simulink model "test"  (R2022b)
settings: Solver=VariableStepAuto  StartTime=0.0  StopTime=20  RelTol=1e-3
values from neighbouring files (symbols this model uses):
  N = 3    [kuka_IMPC_PriController_simulink_initial.m]
undefined symbols (not defined in the file or in its folder): DiscIntNeverNeededParam, exJoint, t_max
libraries: simulink x1, cstblocks x1, cjt_library_models x1
settings Model: Creator=zheng  LastModifiedBy=zheng
settings ModelReferenceCC: EnableRefExpFcnMdlSchedulingChecks=on

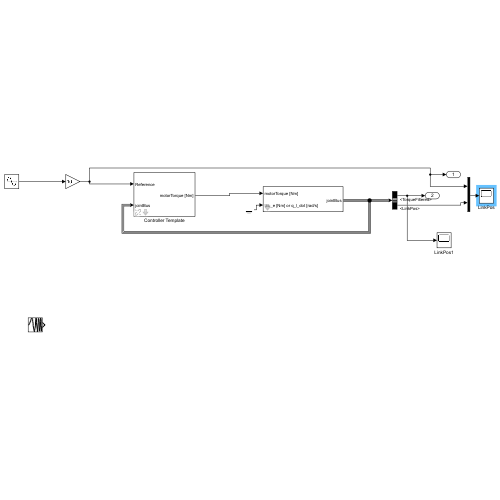
[thumbnail: Simulink's stored preview of the top-level diagram]
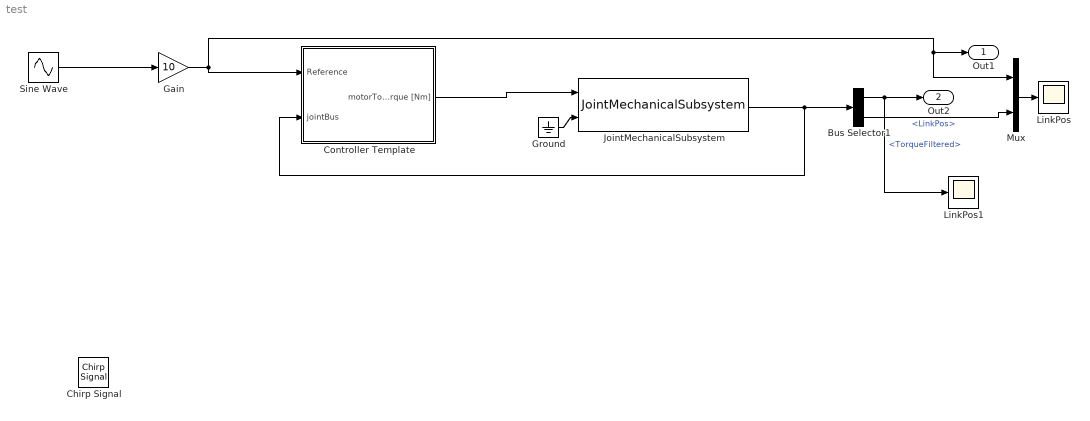
== system test ==
  Bus Selector1 : BusSelector  OutputSignals=TorqueFiltered,LinkPos
  Chirp Signal : simulink/Sources/Chirp Signal  f1=f_min  T=t_max  f2=f_max
  Controller Template : Subsystem  AncestorBlock=cjt_library_controllers/Controllers/Controller Template  mask(CJT Controller Template){jointObj=exJoint}
      mask prompts: jointObj "Joint Object"
      mask help:
      | This is a template block. If you have a controller that you wish to contribute to this library, this block here  represents your interface.
      |
      | Here are the steps to contribute your controller using this template:
      |
      | 1. Copy this block into your development. Disable and break its link to this library. You now have a copy of the interface in your model that is disconnected from the library.
      |
      | 2. Implement your controller within this block. The controller should use no hardcoded values. Wherever you can, access the properties of a CJT joint object. The joint object should be passed to the block through the mask as first parameter (e.g. jointObj).
      |
      | 3. Complete the block mask, so the user can specify all block properties programatically or manually through the mask.
      |
      | 4. Make an example:
      | a) Clean your development model up and convert it into a minimum example that demonstrates the use of your block.
      | b) Create an m-script that configures the required joint object and simulation parameters, runs the model.and displays some results. See existing examples and copy their format.
      | c) Write the documentation of your block.
      |
      | 5. Write a unit test. Look into the unit test directory and open the unit test file for this library. Add a test for your block. A good point to start is your example. Make the test pass.
      |
      | 6. Submit your contribution!
      |
      | Thanks a lot!
      |
      | 7.
      mask init:
      | % Do all the controller related computations here.
      | % Compute gains etc.
      | 
      | % E.g. get linear dynamics matrices first...
      | [A, B, C, I, D, K] = jointObj.getDynamicsMatrices();
      | 
      | % YOUR CODE HERE
      settings: LibrarySourceBlock=cjt_library_controllers/Controllers/Controller Template
      mask Help:
      | This is a template block. If you have a controller that you wish to contribute to this library, this block here  represents your interface.
      | 
      | Here are the steps to contribute your controller using this template:
      | 
      | 1. Copy this block into your development. Disable and break its link to this library. You now have a copy of the interface in your model that is disconnected from the library.
      | 
      | 2. Implement your controller within this block. The controller should use no hardcoded values. Wherever you can, access the properties of a CJT joint object. The joint object should be passed to the block through the mask as first parameter (e.g. jointObj).
      | 
      | 3. Complete the block mask, so the user can specify all block properties programatically or manually through the mask.
      | 
      | 4. Make an example:
      | a) Clean your development model up and convert it into a minimum example that demonstrates the use of your block.
      | b) Create an m-script that configures the required joint object and simulation parameters, runs the model.and displays some results. See existing examples and copy their format.
      | c) Write the documentation of your block.
      | 
      | 5. Write a unit test. Look into the unit test directory and open the unit test file for this library. Add a test for your block. A good point to start is your example. Make the test pass.
      | 
      | 6. Submit your contribution!
      | 
      | Thanks a lot!
  Gain : Gain  Gain=10
  Ground : Ground
  JointMechanicalSubsystem : cjt_library_models/Joint models/JointMechanicalSubsystem  jointObj=exJoint  fc_vel=499  fc_torque=499  input_delay=0  output_delay=0  quantize=on  quantize_bits=19  input_noise_enabled=off  output_noise_enabled=off  var_u=0.12^2  var_y=1.8e-10
  LinkPos : Scope
  LinkPos1 : Scope
  Mux : Mux  Inputs=2
  Sine Wave : Sin  SampleTime=0
  Out1 : Outport
  Out2 : Outport  Port=2
  wires:
  Sine Wave/1 -> Gain/1
  Ground/1 -> JointMechanicalSubsystem/2
  JointMechanicalSubsystem/1 -> Controller Template/2(jointBus), Bus Selector1/1
  Controller Template/1(motorTorque [Nm]) -> JointMechanicalSubsystem/1
  Mux/1 -> LinkPos/1
  Bus Selector1/1 -> LinkPos1/1, Out2/1  "<TorqueFiltered>"
  Gain/1 -> Out1/1, Mux/1, Controller Template/1(Reference)
  Bus Selector1/2 -> Mux/2  "<LinkPos>"

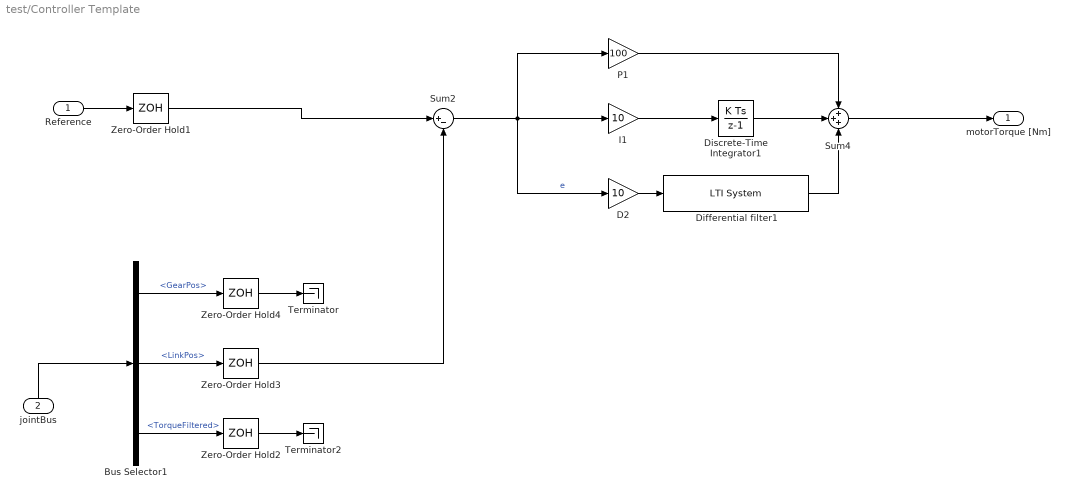
== system test/Controller Template ==
  Reference : Inport
  jointBus : Inport  Port=2
  Bus Selector1 : BusSelector  OutputSignals=GearPos,LinkPos,TorqueFiltered
  D2 : Gain  Gain=10
  Differential filter1 : cstblocks/LTI System  sys=c2d(tf([N 0], [1, N]), jointObj.Ts, 'tustin')  IC=[]
  Discrete-Time Integrator1 : DiscreteIntegrator  SampleTime=-1  ICPrevOutput=DiscIntNeverNeededParam  ICPrevScaledInput=DiscIntNeverNeededParam
  I1 : Gain  Gain=10
  P1 : Gain  Gain=100
  Sum2 : Sum  Inputs=|+-
  Sum4 : Sum  Inputs=+++
  Terminator : Terminator
  Terminator2 : Terminator
  Zero-Order Hold{1..4} (4 alike) : ZeroOrderHold  SampleTime=jointObj.Ts
  motorTorque [Nm] : Outport
  wires:
  Zero-Order Hold4/1 -> Terminator/1
  Zero-Order Hold2/1 -> Terminator2/1
  Sum4/1 -> motorTorque [Nm]/1
  Reference/1 -> Zero-Order Hold1/1
  Bus Selector1/3 -> Zero-Order Hold2/1  "<TorqueFiltered>"
  Bus Selector1/2 -> Zero-Order Hold3/1  "<LinkPos>"
  Bus Selector1/1 -> Zero-Order Hold4/1  "<GearPos>"
  jointBus/1 -> Bus Selector1/1
  Discrete-Time Integrator1/1 -> Sum4/2
  I1/1 -> Discrete-Time Integrator1/1
  Zero-Order Hold1/1 -> Sum2/1
  P1/1 -> Sum4/1
  Differential filter1/1 -> Sum4/3
  Sum2/1 -> D2/1, I1/1, P1/1  "e"
  Zero-Order Hold3/1 -> Sum2/2
  D2/1 -> Differential filter1/1
